simulink model "lab1_model1"  (R2012b)
settings: Solver=ode45  StartTime=0.0  StopTime=10.0  RelTol=1e-3
settings Model: Creator=student-at  LastModifiedBy=student-at

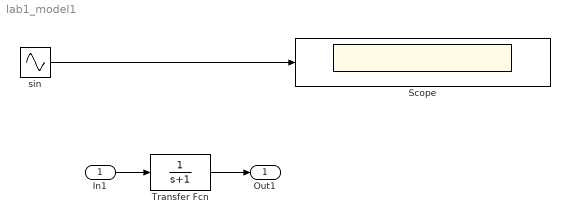
== system lab1_model1 ==
  In1 : Inport
  Scope : Scope
  Transfer Fcn : TransferFcn  Denominator=[1 1]
  sin : Sin  Bias=0.1  Frequency=25  Phase=1  SampleTime=0.01
  Out1 : Outport
  wires:
  sin/1 -> Scope/1
  Transfer Fcn/1 -> Out1/1
  In1/1 -> Transfer Fcn/1
